simulink model "Heli_ID"  (Simulink 6.3)
settings: Solver=ode1  SolverMode=SingleTasking  StartTime=0.0  StopTime=inf  FixedStep=0.001  RelTol=1e-3
values from neighbouring files (symbols this model uses):
  K_CABLE_P = 5    [setip_lab_heli_2d.m]
  K_CABLE_Y = 3    [setip_lab_heli_2d.m]
  K_EC_P = - 2 * pi / ( 4 * 1024 )    (= -0.00153398078789)    [setip_lab_heli_2d.m]
  K_EC_Y = 2 * pi / ( 8 * 1024 )    (= 0.000766990393943)    [setip_lab_heli_2d.m]
  theta_0 = 0    [setip_lab_heli_2d.m]
  VMAX_DAC = 10    [setip_lab_heli_2d.m]
  VMAX_UPM_P = 24    [setip_lab_heli_2d.m]
  VMAX_UPM_Y = 15    [setip_lab_heli_2d.m]
  wcf = 2 * pi * 20    (= 125.663706144)    [setip_lab_heli_2d.m]
  zetaf = 0.85    [setip_lab_heli_2d.m]
undefined symbols (not defined in the file or in its folder): heli_2d_lib, Scopes
libraries: qctools x2, simulink x2, simulink_extras x1
settings Model: LastModifiedBy=localadmin  ExtModeArmWhenConnect=off  BufferReuse=off  StrictBusMsg=None
settings ConfigSet: SimulationMode=external
settings OptimizationCC: BooleanDataType=off  InlineInvariantSignals=on  OptimizeBlockIOStorage=off  BufferReuse=off  ExpressionFolding=off  LocalBlockOutputs=off
settings RTWCC: SystemTargetFile=wincon.tlc  MakeCommand=make_wc  TemplateMakefile=wc_default_tmf  Description=WinCon Target  ProcessScript=wincon_make_rtw_hook
settings STFCustomTargetCC: TargetFcnLib=ansi_tfl_tmw.mat  GenFloatMathFcnCalls=ANSI_C  ModelReferenceCompliant=off  SystemTargetFile=wincon.tlc
settings GRTTargetCC: ModelReferenceCompliant=off  MatFileLogging=off  ExtMode=on  ExtModeTransport=2  ExtModeMexFile=wc_comm
settings CustomProperty: Value=on

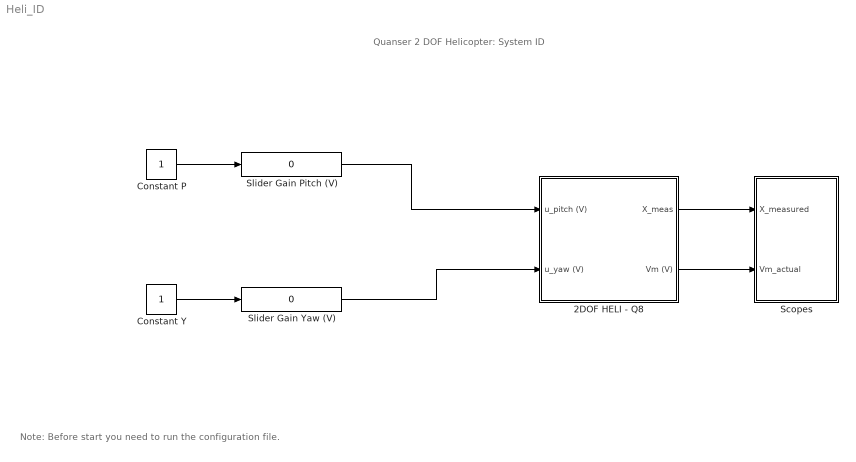
== system Heli_ID ==
  note: Quanser 2 DOF Helicopter:
      | System ID
  note: Note: Before start you need to run the configuration file.
  2DOF HELI - Q8 : Subsystem  AncestorBlock=heli_2d_lib/2DOF HELI - Q8
  Constant P : Constant
  Constant Y : Constant
  Scopes : Subsystem  AncestorBlock=heli_2d_lib/Scopes
  Slider Gain Pitch (V) : simulink/Math Operations/Slider Gain  low=-12  gain=0  high=12
  Slider Gain Yaw (V) : simulink/Math Operations/Slider Gain  low=-12  gain=0  high=12
  wires:
  2DOF HELI - Q8/1(X_meas) -> Scopes/1(X_measured)
  2DOF HELI - Q8/2(Vm (V)) -> Scopes/2(Vm_actual)
  Constant P/1 -> Slider Gain Pitch (V)/1
  Slider Gain Pitch (V)/1 -> 2DOF HELI - Q8/1(u_pitch (V))
  Constant Y/1 -> Slider Gain Yaw (V)/1
  Slider Gain Yaw (V)/1 -> 2DOF HELI - Q8/2(u_yaw (V))

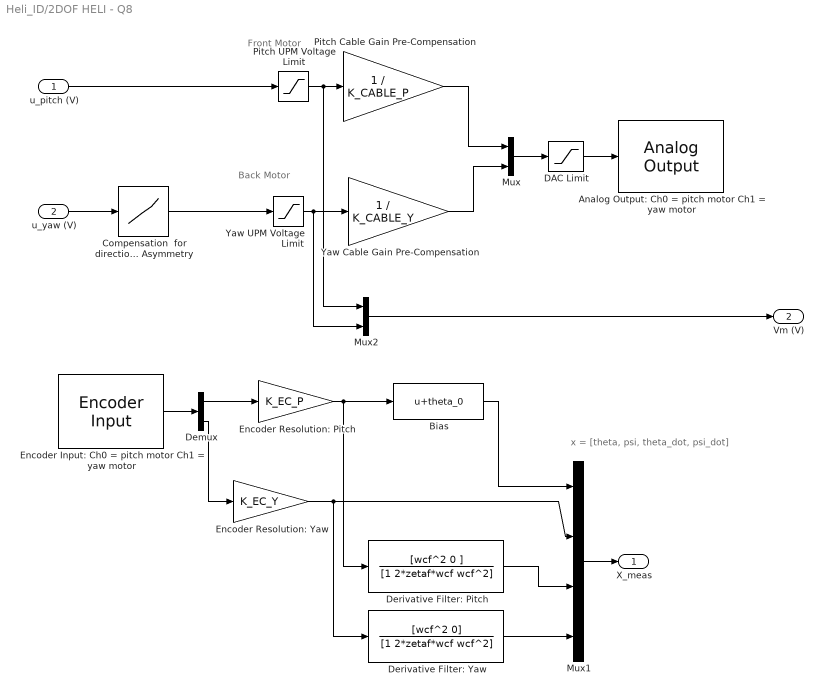
== system Heli_ID/2DOF HELI - Q8 ==
  note: Back Motor
  note: Front Motor
  note: x = [theta, psi, theta_dot, psi_dot]
  u_pitch (V) : Inport
  u_yaw (V) : Inport  Port=2
  Analog Output: Ch0 = pitch motor Ch1 = yaw motor : qctools/Quanser Consulting Q8 Series/Analog Output  boardNumber=0  channels=[0,1]  modesVect=0  rangesVect=10  initialVect=0  finalVect=0  sampleTime=-1  inputVolts=on  simulationOutput=off
  Bias : Bias  Bias=theta_0
  "Compensation  for direction Asymmetry " : Lookup  InputValues="[-[12.5  10 7.5]  0  [7.5 10  12.5 15] ]"  OutputValues="[-[12.5  10 7.5] *.4 0  [7.5 10  12.5 15] ]"
  DAC Limit : Saturate  UpperLimit=VMAX_DAC  LowerLimit=- VMAX_DAC
  Demux : Demux  Outputs=2
  Derivative Filter: Pitch : TransferFcn  Numerator=[wcf^2 0 ]  Denominator=[1 2*zetaf*wcf wcf^2]
  Derivative Filter: Yaw : TransferFcn  Numerator=[wcf^2 0]  Denominator=[1 2*zetaf*wcf wcf^2]
  Encoder Input: Ch0 = pitch motor Ch1 = yaw motor : qctools/Quanser Consulting Q8 Series/Encoder Input  boardNumber=0  channels=[0,1]  initial=0  preserveCounts=off  sampleTime=default_sample_time  quadratureStr=4X  modeStr=Normal  flagString=FLG1 is IDX and FLG2 is E  prescale=1  frequency=16666666.6667  bcd=off  enableIndex=on  synchronousIndex=on  indexPolarity=on  reloadOnIndex=off  simulationInput=off
  "Encoder Resolution: Pitch " : Gain  Gain=K_EC_P
  Encoder Resolution: Yaw : Gain  Gain=K_EC_Y
  Mux : Mux  Inputs=2
  Mux1 : Mux
  Mux2 : Mux  Inputs=2
  Pitch Cable Gain Pre-Compensation : Gain  Gain=1 / K_CABLE_P  SaturateOnIntegerOverflow=on
  Pitch UPM Voltage Limit : Saturate  UpperLimit=VMAX_UPM_P  LowerLimit=- VMAX_UPM_P
  Yaw Cable Gain Pre-Compensation : Gain  Gain=1 / K_CABLE_Y  SaturateOnIntegerOverflow=on
  Yaw UPM Voltage Limit : Saturate  UpperLimit=VMAX_UPM_Y  LowerLimit=- VMAX_UPM_Y
  X_meas : Outport
  Vm (V) : Outport  Port=2
  wires:
  Encoder Resolution: Yaw/1 -> Mux1/2, Derivative Filter: Yaw/1
  Mux2/1 -> Vm (V)/1
  Yaw Cable Gain Pre-Compensation/1 -> Mux/2
  Pitch Cable Gain Pre-Compensation/1 -> Mux/1
  Mux1/1 -> X_meas/1
  u_pitch (V)/1 -> Pitch UPM Voltage Limit/1
  Yaw UPM Voltage Limit/1 -> Mux2/2, Yaw Cable Gain Pre-Compensation/1
  Pitch UPM Voltage Limit/1 -> Mux2/1, Pitch Cable Gain Pre-Compensation/1
  DAC Limit/1 -> Analog Output: Ch0 = pitch motor Ch1 = yaw motor/1
  Mux/1 -> DAC Limit/1
  Demux/1 -> "Encoder Resolution: Pitch "/1
  "Encoder Resolution: Pitch "/1 -> Bias/1, Derivative Filter: Pitch/1
  Encoder Input: Ch0 = pitch motor Ch1 = yaw motor/1 -> Demux/1
  Demux/2 -> Encoder Resolution: Yaw/1
  Bias/1 -> Mux1/1
  Derivative Filter: Pitch/1 -> Mux1/3
  Derivative Filter: Yaw/1 -> Mux1/4
  "Compensation  for direction Asymmetry "/1 -> Yaw UPM Voltage Limit/1
  u_yaw (V)/1 -> "Compensation  for direction Asymmetry "/1

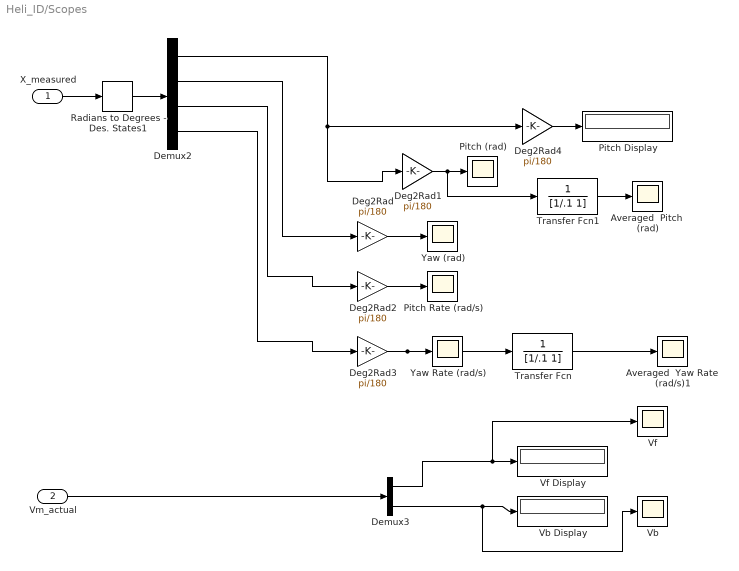
== system Heli_ID/Scopes ==
  X_measured : Inport
  Vm_actual : Inport  Port=2
  Averaged  Pitch  (rad) : Scope
      settings: TickLabels=on  TimeRange=1.000000  YMin=-250  YMax=250  SaveName=ScopeData5  DataFormat=Array
  Averaged  Yaw Rate  (rad/s)1 : Scope
      settings: TickLabels=on  TimeRange=1.000000  YMin=-250  YMax=250  SaveName=ScopeData4  DataFormat=Array
  Deg2Rad{,1..4} (5 alike) : Gain  Gain=pi/180
  Demux2 : Demux
  Demux3 : Demux  Outputs=2
  Pitch (rad) : Scope
      settings: TickLabels=on  TimeRange=50  YMin=-15  YMax=15  DataFormat=Array
  Pitch Display : Display
  Pitch Rate (rad/s) : Scope
      settings: TickLabels=on  TimeRange=1.000000  YMin=-250  YMax=250  SaveName=ScopeData2  DataFormat=Array
  Radians to Degrees - Des. States1 : simulink_extras/Transformations/Radians to Degrees
  Transfer Fcn : TransferFcn  Denominator=[1/.1 1]
  Transfer Fcn1 : TransferFcn  Denominator=[1/.1 1]
  Vb : Scope
      settings: TickLabels=on  TimeRange=1.000000  YMin=-250  YMax=250  DataFormat=Array
  "Vb Display " : Display
  Vf : Scope
      settings: TickLabels=on  TimeRange=1.000000  YMin=-250  YMax=250  DataFormat=Array
  Vf Display : Display
  Yaw (rad) : Scope
      settings: TickLabels=on  TimeRange=50  YMin=-5.5  YMax=5.5  DataFormat=Array
  Yaw Rate (rad/s) : Scope
      settings: TickLabels=on  TimeRange=1.000000  YMin=-250  YMax=250  SaveName=ScopeData3  DataFormat=Array
  wires:
  Demux2/2 -> Deg2Rad/1
  Demux2/3 -> Deg2Rad2/1
  Demux2/4 -> Deg2Rad3/1
  X_measured/1 -> Radians to Degrees - Des. States1/1
  Vm_actual/1 -> Demux3/1
  Radians to Degrees - Des. States1/1 -> Demux2/1
  Deg2Rad/1 -> Yaw (rad)/1
  Deg2Rad3/1 -> Yaw Rate (rad/s)/1, Transfer Fcn/1
  Deg2Rad2/1 -> Pitch Rate (rad/s)/1
  Deg2Rad1/1 -> Pitch (rad)/1, Transfer Fcn1/1
  Demux3/1 -> Vf Display/1, Vf/1
  Demux3/2 -> "Vb Display "/1, Vb/1
  Demux2/1 -> Deg2Rad4/1, Deg2Rad1/1
  Deg2Rad4/1 -> Pitch Display/1
  Transfer Fcn/1 -> Averaged  Yaw Rate  (rad/s)1/1
  Transfer Fcn1/1 -> Averaged  Pitch  (rad)/1
